simulink model "TopModel"  (R2026a)
settings: Solver=FixedStepAuto  EnableMultiTasking=on
undefined symbols (not defined in the file or in its folder): D1, D2, m, n, P
libraries: procinterlib x2, proctasklib x2
settings Model: Creator=ttichy  LastModifiedBy=chmurski
settings SolverCC: PositivePriorityOrder=on
settings OptimizationCC: StrengthReduction=on  MaxStackSize=2048
settings HardwareCC: ProdLargestAtomicInteger=Long  ProdHWDeviceType=Infineon->TriCore  HardwareBoardFeatureSet=SoCBlockset
settings RTWCC: SystemTargetFile=ert.tlc  HardwareBoard=Infineon AURIX TC4x  TLCOptions=-aInlineSetEventsForThisBaseRateFcn=TLC_FALSE -aSuppressMultiTaskScheduler=TLC_FALSE -aRateBasedStepFcn=1  GenerateReport=on  Toolchain=TASKING SmartCode for TriCore  BuildConfiguration=Specify  IncludeHyperlinkInReport=on  LaunchReport=on  GenerateTraceInfo=on  GenerateTraceReport=on  GenerateTraceReportSl=on  GenerateTraceReportSf=on  GenerateTraceReportEml=on  GenerateCodeMetricsReport=on  GenerateCodeReplacementReport=on  Description=Embedded Coder
settings CodeAppCC: MaxIdLength=256.0
settings ERTTargetCC: ExtModeTransport=3.0  ERTFilePackagingFormat=Compact  DynamicArrayContainerType=coder::array  SupportAbsoluteTime=off  SupportNonFinite=off

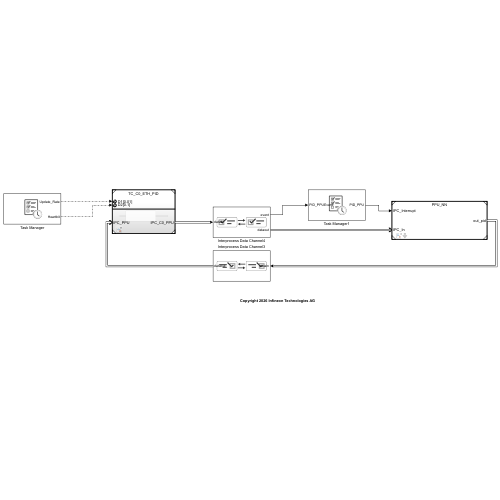
[thumbnail: Simulink's stored preview of the top-level diagram]
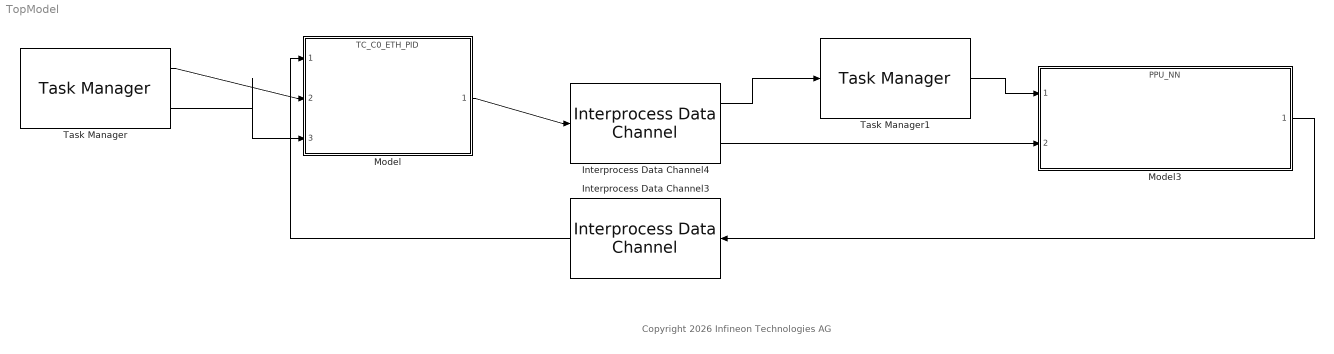
== system TopModel ==
  note: Copyright 2026 Infineon Technologies AG
  Interprocess Data Channel3 : procinterlib/Interprocess Data Channel  NumBuffers=1  PropagationDelay=3e-6  ShowEventPort=off  ShowNumUsedBuffers=off  ShowBufferOverwritten=off
      settings: LibrarySourceBlock=aurixtc4xlib/Test Bench Blocks/Interprocess Data Channel
  Interprocess Data Channel4 : procinterlib/Interprocess Data Channel  NumBuffers=1  PropagationDelay=3e-6  ShowEventPort=on  ShowNumUsedBuffers=off  ShowBufferOverwritten=off
      settings: LibrarySourceBlock=aurixtc4xlib/Test Bench Blocks/Interprocess Data Channel
  Model : ModelReference  InputPortMessageModes=m,n,n  OutputPortMessageModes=m  ModelNameDialog=TC_C0_ETH_PID.slx  SimulationMode=Normal  ScheduleRates=on  CachedPortDiscreteRates=[0.01;0.1]  ModelEventPortInfo=P:D1[0.01][0][0],P:D2[0.1][0][0]  ModelReferenceVersion=5.29
  Model3 : ModelReference  InputPortMessageModes=n,m  OutputPortMessageModes=m  ModelNameDialog=PPU_NN.slx  SimulationMode=Normal  CachedPortDiscreteRates=[0.01]  ModelReferenceVersion=5.8
  Task Manager : proctasklib/Task Manager  AllTaskData="[{\"taskName\":\"Update_Rate\",\"taskType\":\"Timer-driven\",\"taskEvent\":\"<empty>\",\"taskPeriod\":\"0.01\",\"taskPriority\":\"10\",\"coreSelection\":\"Specified core\",\"coreNum\":\"0\",\"dropOverranTasks\":false,\"playbackRecorded\":false,\"diagnosticsFile\":\"\",\"taskDurationSource\":\"Dialog\",\"taskDuration\":1E-6,\"taskDurationDeviation\":0,\"logExecutionData\":true,\"logDroppedTasks\":false,\"version\":\"2.6\",\"taskDurationData\":{\"percent\":\"100\",\"mean\":\"1e-06\",\"dev\":\"0\",\"min\":\"1e-06\",\"max\":\"1e-06\"},\"taskEventSource\":\"Internal\",\"taskEventSourceAssignmentType\":\"AutoAssigned\",\"taskEventSourceType\":\"Unspecified\",\"taskEventGroup\":\"Unspecified\",\"taskEventInterrupt\":\"Unspecified\",\"taskEventOrder\":1,\"taskDisablePremption\":false,\"taskClearInterruptFlagsAtEndOfEvent\":false},{\"taskName\":\"Heartbit\",\"taskType\":\"Timer-driven\",\"taskEvent\":\"HeartbitEvent\",\"taskPeriod\":\"0.1\",\"taskPriority\":\"50\",\"coreSelection\":\"Specified core\",\"coreNum\":\"0\",\"dropOverranTasks\":false,\"playbackRecorded\":false,\"diagnosticsFile\":\"\",\"taskDurationSource\":\"Dialog\",\"taskDuration\":1E-6,\"taskDurationDeviation\":0,\"logExecutionData\":true,\"logDroppedTasks\":false,\"version\":\"2.6\",\"taskDurationData\":{\"percent\":\"100\",\"mean\":\"1e-06\",\"dev\":\"0\",\"min\":\"1e-06\",\"max\":\"1e-06\"},\"taskEventSource\":\"Internal\",\"taskEventSourceAssignmentType\":\"AutoAssigned\",\"taskEventSourceType\":\"Unspecified\",\"taskEventGroup\":\"Unspecified\",\"taskEventInterrupt\":\"Unspecified\",\"taskEventOrder\":1,\"taskDisablePremption\":false,\"taskClearInterruptFlagsAtEndOfEvent\":false}]"  EnableTaskSimulation=off  StreamToSDI=on  WriteToFile=off  OverwriteFile=off  SupportEventPorts=on  UseScheduleEditor=off  CustomizationInfo=''
      settings: LibrarySourceBlock=aurixtc4xlib/Scheduling/Task Manager
  Task Manager1 : proctasklib/Task Manager  AllTaskData="{\"taskName\":\"PID_PPU\",\"taskType\":\"Event-driven\",\"taskEvent\":\"PID_PPUEvent\",\"taskPeriod\":\"0.01\",\"taskPriority\":\"50\",\"coreSelection\":\"Specified core\",\"coreNum\":\"0\",\"dropOverranTasks\":false,\"playbackRecorded\":false,\"diagnosticsFile\":\"\",\"taskDurationSource\":\"Dialog\",\"taskDuration\":1E-6,\"taskDurationDeviation\":0,\"logExecutionData\":true,\"logDroppedTasks\":false,\"version\":\"2.6\",\"taskDurationData\":{\"percent\":\"100\",\"mean\":\"1e-06\",\"dev\":\"0\",\"min\":\"1e-06\",\"max\":\"1e-06\"},\"taskEventSource\":\"Default event\",\"taskEventSourceAssignmentType\":\"ManuallyAssigned\",\"taskEventSourceType\":\"Unspecified\",\"taskEventGroup\":\"IPC\",\"taskEventInterrupt\":\"IPC_Interrupt_Stanley_PPU\",\"taskEventOrder\":1,\"taskDisablePremption\":false,\"taskClearInterruptFlagsAtEndOfEvent\":false}"  EnableTaskSimulation=on  StreamToSDI=on  WriteToFile=off  OverwriteFile=off  SupportEventPorts=on  UseScheduleEditor=off  CustomizationInfo=''
      settings: LibrarySourceBlock=aurixtc4xlib/Scheduling/Task Manager
  wires:
  Model/1 -> Interprocess Data Channel4/1
  Interprocess Data Channel3/1 -> Model/1
  Task Manager/2 -> Model/3
  Task Manager/1 -> Model/2
  Model3/1 -> Interprocess Data Channel3/1
  Interprocess Data Channel4/2 -> Model3/2
  Interprocess Data Channel4/1 -> Task Manager1/1
  Task Manager1/1 -> Model3/1
